simulink model "case5"  (R2024b)
settings: Solver=FixedStepAuto  StartTime=0  StopTime=1  FixedStep=1e-7  RelTol=1e-3
values from neighbouring files (symbols this model uses):
  SG_D_1_D = 0.01056    [IEEE9_case_parameters.m]    (also in case1_parameters.m; case2_parameters.m; case3_parameters.m; case4_parameters.m)
  SG_D_1_EnableSaturation = 0    [IEEE9_case_parameters.m]    (also in case1_parameters.m; case2_parameters.m; case3_parameters.m; case4_parameters.m)
  SG_D_1_f0 = 60    [IEEE9_case_parameters.m]    (also in case1_parameters.m; case2_parameters.m; case3_parameters.m; case4_parameters.m)
  SG_D_1_H = 7.5    [IEEE9_case_parameters.m]    (also in case1_parameters.m; case2_parameters.m; case3_parameters.m; case4_parameters.m)
  SG_D_1_K_A = 20    [IEEE9_case_parameters.m]    (also in case1_parameters.m; case2_parameters.m; case3_parameters.m; case4_parameters.m)
  SG_D_1_K_E = 1.000000e+1    (= 10)    [IEEE9_case_parameters.m]    (also in case1_parameters.m; case2_parameters.m; case3_parameters.m; case4_parameters.m)
  SG_D_1_K_F = 2.363    [IEEE9_case_parameters.m]    (also in case1_parameters.m; case2_parameters.m; case3_parameters.m; case4_parameters.m)
  SG_D_1_K_s = 0.5    [IEEE9_case_parameters.m]    (also in case1_parameters.m = 5; case2_parameters.m = 5; case3_parameters.m = 5; case4_parameters.m = 5)
  SG_D_1_R_a = 0.001088    [IEEE9_case_parameters.m]    (also in case1_parameters.m; case2_parameters.m; case3_parameters.m; case4_parameters.m)
  SG_D_1_S_A = 1    [IEEE9_case_parameters.m]    (also in case1_parameters.m; case2_parameters.m; case3_parameters.m; case4_parameters.m)
  SG_D_1_S_B = 0.103    [IEEE9_case_parameters.m]    (also in case1_parameters.m; case2_parameters.m; case3_parameters.m; case4_parameters.m)
  SG_D_1_S_N = 10.659857    [IEEE9_case_parameters.m]    (also in case1_parameters.m; case2_parameters.m; case3_parameters.m; case4_parameters.m)
  SG_D_1_SpeedPara = 200    [IEEE9_case_parameters.m]    (also in case1_parameters.m; case2_parameters.m; case3_parameters.m; case4_parameters.m)
  SG_D_1_T_0 = 0.720173    [IEEE9_case_parameters.m]    (also in case1_parameters.m = 0.755522; case2_parameters.m = 0.808931; case3_parameters.m = 0.869402; case4_parameters.m = 0.729316)
  SG_D_1_T_1 = 0.3    [IEEE9_case_parameters.m]    (also in case1_parameters.m; case2_parameters.m; case3_parameters.m; case4_parameters.m)
  SG_D_1_T_2 = 0.05    [IEEE9_case_parameters.m]    (also in case1_parameters.m; case2_parameters.m; case3_parameters.m; case4_parameters.m)
  SG_D_1_T_3 = 0.02    [IEEE9_case_parameters.m]    (also in case1_parameters.m; case2_parameters.m; case3_parameters.m; case4_parameters.m)
  SG_D_1_T_4 = 0.005    [IEEE9_case_parameters.m]    (also in case1_parameters.m; case2_parameters.m; case3_parameters.m; case4_parameters.m)
  SG_D_1_T_A = 0.02    [IEEE9_case_parameters.m]    (also in case1_parameters.m; case2_parameters.m; case3_parameters.m; case4_parameters.m)
  SG_D_1_T_dd = 8.000000e+0    (= 8)    [IEEE9_case_parameters.m]    (also in case1_parameters.m; case2_parameters.m; case3_parameters.m; case4_parameters.m)
  SG_D_1_T_ddd = 0.04    [IEEE9_case_parameters.m]    (also in case1_parameters.m; case2_parameters.m; case3_parameters.m; case4_parameters.m)
  SG_D_1_T_E = 0.314    [IEEE9_case_parameters.m]    (also in case1_parameters.m; case2_parameters.m; case3_parameters.m; case4_parameters.m)
  SG_D_1_T_F = 0.35    [IEEE9_case_parameters.m]    (also in case1_parameters.m; case2_parameters.m; case3_parameters.m; case4_parameters.m)
  SG_D_1_T_qd = 0.8    [IEEE9_case_parameters.m]    (also in case1_parameters.m; case2_parameters.m; case3_parameters.m; case4_parameters.m)
  SG_D_1_T_qdd = 0.02    [IEEE9_case_parameters.m]    (also in case1_parameters.m; case2_parameters.m; case3_parameters.m; case4_parameters.m)
  SG_D_1_T_speed = 0.1    [IEEE9_case_parameters.m]    (also in case1_parameters.m = 200; case2_parameters.m = 200; case3_parameters.m = 200; case4_parameters.m = 200)
  SG_D_1_T_w = 0.5    [IEEE9_case_parameters.m]    (also in case1_parameters.m; case2_parameters.m; case3_parameters.m; case4_parameters.m)
  SG_D_1_V_ref = 1.990276    [IEEE9_case_parameters.m]    (also in case1_parameters.m = 2.042296; case2_parameters.m = 2.051388; case3_parameters.m = 2.089584; case4_parameters.m = 2.01845)
  SG_D_1_w_ref = 376.991118    [IEEE9_case_parameters.m]    (also in case1_parameters.m; case2_parameters.m; case3_parameters.m; case4_parameters.m)
  SG_D_1_wb = 6.000000e+1    (= 60)    [IEEE9_case_parameters.m]    (also in case1_parameters.m; case2_parameters.m; case3_parameters.m; case4_parameters.m)
  SG_D_1_x_d = 1.9    [IEEE9_case_parameters.m]    (also in case1_parameters.m; case2_parameters.m; case3_parameters.m; case4_parameters.m)
  SG_D_1_x_dd = 0.302    [IEEE9_case_parameters.m]    (also in case1_parameters.m; case2_parameters.m; case3_parameters.m; case4_parameters.m)
  SG_D_1_x_ddd = 0.204    [IEEE9_case_parameters.m]    (also in case1_parameters.m; case2_parameters.m; case3_parameters.m; case4_parameters.m)
  SG_D_1_x_l = 0.05    [IEEE9_case_parameters.m]    (also in case1_parameters.m; case2_parameters.m; case3_parameters.m; case4_parameters.m)
  SG_D_1_x_q = 1.3    [IEEE9_case_parameters.m]    (also in case1_parameters.m; case2_parameters.m; case3_parameters.m; case4_parameters.m)
  SG_D_1_x_qd = 0.5    [IEEE9_case_parameters.m]    (also in case1_parameters.m; case2_parameters.m; case3_parameters.m; case4_parameters.m)
  SG_D_1_x_qdd = 0.3    [IEEE9_case_parameters.m]    (also in case1_parameters.m; case2_parameters.m; case3_parameters.m; case4_parameters.m)
  SG_D_2_D = 0.02    [IEEE9_case_parameters.m]    (also in case1_parameters.m; case2_parameters.m; case3_parameters.m; case4_parameters.m)
  SG_D_2_EnableSaturation = 0    [IEEE9_case_parameters.m]    (also in case1_parameters.m; case2_parameters.m; case3_parameters.m; case4_parameters.m)
  SG_D_2_f0 = 60    [IEEE9_case_parameters.m]    (also in case1_parameters.m; case2_parameters.m; case3_parameters.m; case4_parameters.m)
  SG_D_2_H = 8.000000e+0    (= 8)    [IEEE9_case_parameters.m]    (also in case1_parameters.m; case2_parameters.m; case3_parameters.m; case4_parameters.m)
  SG_D_2_K_A = 20    [IEEE9_case_parameters.m]    (also in case1_parameters.m; case2_parameters.m; case3_parameters.m; case4_parameters.m)
  SG_D_2_K_E = 1.000000e+1    (= 10)    [IEEE9_case_parameters.m]    (also in case1_parameters.m; case2_parameters.m; case3_parameters.m; case4_parameters.m)
  SG_D_2_K_F = 2.363    [IEEE9_case_parameters.m]    (also in case1_parameters.m; case2_parameters.m; case3_parameters.m; case4_parameters.m)
  SG_D_2_K_s = 0.5    [IEEE9_case_parameters.m]    (also in case1_parameters.m = 4; case2_parameters.m = 4; case3_parameters.m = 4; case4_parameters.m = 4)
  SG_D_2_R_a = 0.001088    [IEEE9_case_parameters.m]    (also in case1_parameters.m; case2_parameters.m; case3_parameters.m; case4_parameters.m)
  SG_D_2_S_A = 1    [IEEE9_case_parameters.m]    (also in case1_parameters.m; case2_parameters.m; case3_parameters.m; case4_parameters.m)
  SG_D_2_S_B = 0.103    [IEEE9_case_parameters.m]    (also in case1_parameters.m; case2_parameters.m; case3_parameters.m; case4_parameters.m)
  SG_D_2_S_N = 10.659857    [IEEE9_case_parameters.m]    (also in case1_parameters.m; case2_parameters.m; case3_parameters.m; case4_parameters.m)
  SG_D_2_SpeedPara = 200    [IEEE9_case_parameters.m]    (also in case1_parameters.m; case2_parameters.m; case3_parameters.m; case4_parameters.m)
  SG_D_2_T_0 = 1.632913    [IEEE9_case_parameters.m]    (also in case1_parameters.m = 1.632925; case2_parameters.m = 1.632915; case3_parameters.m = 1.632914; case4_parameters.m = 1.632927)
  SG_D_2_T_1 = 0.2    [IEEE9_case_parameters.m]    (also in case1_parameters.m; case2_parameters.m; case3_parameters.m; case4_parameters.m)
  SG_D_2_T_2 = 0.05    [IEEE9_case_parameters.m]    (also in case1_parameters.m; case2_parameters.m; case3_parameters.m; case4_parameters.m)
  SG_D_2_T_3 = 0.02    [IEEE9_case_parameters.m]    (also in case1_parameters.m; case2_parameters.m; case3_parameters.m; case4_parameters.m)
  SG_D_2_T_4 = 0.005    [IEEE9_case_parameters.m]    (also in case1_parameters.m; case2_parameters.m; case3_parameters.m; case4_parameters.m)
  SG_D_2_T_A = 0.02    [IEEE9_case_parameters.m]    (also in case1_parameters.m; case2_parameters.m; case3_parameters.m; case4_parameters.m)
  SG_D_2_T_dd = 7.9    [IEEE9_case_parameters.m]    (also in case1_parameters.m; case2_parameters.m; case3_parameters.m; case4_parameters.m)
  SG_D_2_T_ddd = 0.04    [IEEE9_case_parameters.m]    (also in case1_parameters.m; case2_parameters.m; case3_parameters.m; case4_parameters.m)
  SG_D_2_T_E = 0.314    [IEEE9_case_parameters.m]    (also in case1_parameters.m; case2_parameters.m; case3_parameters.m; case4_parameters.m)
  SG_D_2_T_F = 0.35    [IEEE9_case_parameters.m]    (also in case1_parameters.m; case2_parameters.m; case3_parameters.m; case4_parameters.m)
  SG_D_2_T_qd = 0.8    [IEEE9_case_parameters.m]    (also in case1_parameters.m; case2_parameters.m; case3_parameters.m; case4_parameters.m)
  SG_D_2_T_qdd = 0.015    [IEEE9_case_parameters.m]    (also in case1_parameters.m; case2_parameters.m; case3_parameters.m; case4_parameters.m)
  SG_D_2_T_speed = 0.1    [IEEE9_case_parameters.m]    (also in case1_parameters.m = 150; case2_parameters.m = 150; case3_parameters.m = 150; case4_parameters.m = 150)
  SG_D_2_T_w = 0.35    [IEEE9_case_parameters.m]    (also in case1_parameters.m; case2_parameters.m; case3_parameters.m; case4_parameters.m)
  SG_D_2_V_ref = 2.58547    [IEEE9_case_parameters.m]    (also in case1_parameters.m = 2.597896; case2_parameters.m = 2.587136; case3_parameters.m = 2.586042; case4_parameters.m = 2.599679)
  SG_D_2_w_ref = 376.991118    [IEEE9_case_parameters.m]    (also in case1_parameters.m; case2_parameters.m; case3_parameters.m; case4_parameters.m)
  SG_D_2_wb = 6.000000e+1    (= 60)    [IEEE9_case_parameters.m]    (also in case1_parameters.m; case2_parameters.m; case3_parameters.m; case4_parameters.m)
  SG_D_2_x_d = 1.8    [IEEE9_case_parameters.m]    (also in case1_parameters.m; case2_parameters.m; case3_parameters.m; case4_parameters.m)
  SG_D_2_x_dd = 0.302    [IEEE9_case_parameters.m]    (also in case1_parameters.m; case2_parameters.m; case3_parameters.m; case4_parameters.m)
  SG_D_2_x_ddd = 0.204    [IEEE9_case_parameters.m]    (also in case1_parameters.m; case2_parameters.m; case3_parameters.m; case4_parameters.m)
  SG_D_2_x_l = 0.05    [IEEE9_case_parameters.m]    (also in case1_parameters.m; case2_parameters.m; case3_parameters.m; case4_parameters.m)
  SG_D_2_x_q = 1.25    [IEEE9_case_parameters.m]    (also in case1_parameters.m; case2_parameters.m; case3_parameters.m; case4_parameters.m)
  SG_D_2_x_qd = 0.5    [IEEE9_case_parameters.m]    (also in case1_parameters.m; case2_parameters.m; case3_parameters.m; case4_parameters.m)
  SG_D_2_x_qdd = 0.3    [IEEE9_case_parameters.m]    (also in case1_parameters.m; case2_parameters.m; case3_parameters.m; case4_parameters.m)
  SG_D_3_D = 0.02    [IEEE9_case_parameters.m]    (also in case1_parameters.m; case2_parameters.m; case3_parameters.m; case4_parameters.m)
  SG_D_3_EnableSaturation = 0    [IEEE9_case_parameters.m]    (also in case1_parameters.m; case2_parameters.m; case3_parameters.m; case4_parameters.m)
  SG_D_3_f0 = 60    [IEEE9_case_parameters.m]    (also in case1_parameters.m; case2_parameters.m; case3_parameters.m; case4_parameters.m)
  SG_D_3_H = 7.7    [IEEE9_case_parameters.m]    (also in case1_parameters.m; case2_parameters.m; case3_parameters.m; case4_parameters.m)
  SG_D_3_K_A = 20    [IEEE9_case_parameters.m]    (also in case1_parameters.m; case2_parameters.m; case3_parameters.m; case4_parameters.m)
  SG_D_3_K_E = 1.000000e+1    (= 10)    [IEEE9_case_parameters.m]    (also in case1_parameters.m; case2_parameters.m; case3_parameters.m; case4_parameters.m)
  SG_D_3_K_F = 2.363    [IEEE9_case_parameters.m]    (also in case1_parameters.m; case2_parameters.m; case3_parameters.m; case4_parameters.m)
  SG_D_3_K_s = 0.2    [IEEE9_case_parameters.m]    (also in case1_parameters.m = 2; case2_parameters.m = 2; case3_parameters.m = 2; case4_parameters.m = 2)
  SG_D_3_R_a = 0.001088    [IEEE9_case_parameters.m]    (also in case1_parameters.m; case2_parameters.m; case3_parameters.m; case4_parameters.m)
  SG_D_3_S_A = 1    [IEEE9_case_parameters.m]    (also in case1_parameters.m; case2_parameters.m; case3_parameters.m; case4_parameters.m)
  SG_D_3_S_B = 0.103    [IEEE9_case_parameters.m]    (also in case1_parameters.m; case2_parameters.m; case3_parameters.m; case4_parameters.m)
  SG_D_3_S_N = 10.659857    [IEEE9_case_parameters.m]    (also in case1_parameters.m; case2_parameters.m; case3_parameters.m; case4_parameters.m)
  SG_D_3_SpeedPara = 200    [IEEE9_case_parameters.m]    (also in case1_parameters.m; case2_parameters.m; case3_parameters.m; case4_parameters.m)
  SG_D_3_T_0 = 0.850788    [IEEE9_case_parameters.m]    (also in case1_parameters.m = 0.850786; case2_parameters.m = 0.850787; case3_parameters.m; case4_parameters.m = 0.850786)
  SG_D_3_T_1 = 0.2    [IEEE9_case_parameters.m]    (also in case1_parameters.m; case2_parameters.m; case3_parameters.m; case4_parameters.m)
  SG_D_3_T_2 = 0.05    [IEEE9_case_parameters.m]    (also in case1_parameters.m; case2_parameters.m; case3_parameters.m; case4_parameters.m)
  SG_D_3_T_3 = 0.02    [IEEE9_case_parameters.m]    (also in case1_parameters.m; case2_parameters.m; case3_parameters.m; case4_parameters.m)
  SG_D_3_T_4 = 0.005    [IEEE9_case_parameters.m]    (also in case1_parameters.m; case2_parameters.m; case3_parameters.m; case4_parameters.m)
  SG_D_3_T_A = 0.02    [IEEE9_case_parameters.m]    (also in case1_parameters.m; case2_parameters.m; case3_parameters.m; case4_parameters.m)
  SG_D_3_T_dd = 8.1    [IEEE9_case_parameters.m]    (also in case1_parameters.m; case2_parameters.m; case3_parameters.m; case4_parameters.m)
  SG_D_3_T_ddd = 0.04    [IEEE9_case_parameters.m]    (also in case1_parameters.m; case2_parameters.m; case3_parameters.m; case4_parameters.m)
  SG_D_3_T_E = 0.314    [IEEE9_case_parameters.m]    (also in case1_parameters.m; case2_parameters.m; case3_parameters.m; case4_parameters.m)
  SG_D_3_T_F = 0.35    [IEEE9_case_parameters.m]    (also in case1_parameters.m; case2_parameters.m; case3_parameters.m; case4_parameters.m)
  SG_D_3_T_qd = 0.8    [IEEE9_case_parameters.m]    (also in case1_parameters.m; case2_parameters.m; case3_parameters.m; case4_parameters.m)
  SG_D_3_T_qdd = 0.015    [IEEE9_case_parameters.m]    (also in case1_parameters.m; case2_parameters.m; case3_parameters.m; case4_parameters.m)
  SG_D_3_T_speed = 0.1    [IEEE9_case_parameters.m]    (also in case1_parameters.m = 180; case2_parameters.m = 180; case3_parameters.m = 180; case4_parameters.m = 180)
  SG_D_3_T_w = 0.4    [IEEE9_case_parameters.m]    (also in case1_parameters.m; case2_parameters.m; case3_parameters.m; case4_parameters.m)
  SG_D_3_V_ref = 1.892727    [IEEE9_case_parameters.m]    (also in case1_parameters.m = 1.906439; case2_parameters.m = 1.895535; case3_parameters.m = 1.892105; case4_parameters.m = 1.906598)
  SG_D_3_w_ref = 376.991118    [IEEE9_case_parameters.m]    (also in case1_parameters.m; case2_parameters.m; case3_parameters.m; case4_parameters.m)
  SG_D_3_wb = 6.000000e+1    (= 60)    [IEEE9_case_parameters.m]    (also in case1_parameters.m; case2_parameters.m; case3_parameters.m; case4_parameters.m)
  SG_D_3_x_d = 1.85    [IEEE9_case_parameters.m]    (also in case1_parameters.m; case2_parameters.m; case3_parameters.m; case4_parameters.m)
  SG_D_3_x_dd = 0.302    [IEEE9_case_parameters.m]    (also in case1_parameters.m; case2_parameters.m; case3_parameters.m; case4_parameters.m)
  SG_D_3_x_ddd = 0.204    [IEEE9_case_parameters.m]    (also in case1_parameters.m; case2_parameters.m; case3_parameters.m; case4_parameters.m)
  SG_D_3_x_l = 0.05    [IEEE9_case_parameters.m]    (also in case1_parameters.m; case2_parameters.m; case3_parameters.m; case4_parameters.m)
  SG_D_3_x_q = 1.2    [IEEE9_case_parameters.m]    (also in case1_parameters.m; case2_parameters.m; case3_parameters.m; case4_parameters.m)
  SG_D_3_x_qd = 0.5    [IEEE9_case_parameters.m]    (also in case1_parameters.m; case2_parameters.m; case3_parameters.m; case4_parameters.m)
  SG_D_3_x_qdd = 0.3    [IEEE9_case_parameters.m]    (also in case1_parameters.m; case2_parameters.m; case3_parameters.m; case4_parameters.m)
(part 3 of 12)

== system case5/AC_1/d_id_load_7_block ==
  note: d_id_load_7 in case5
      | $376.991118430775\,\mathrm{iq}_{\mathrm{load},7}-1031.50171752067\,\mathrm{id}_{\mathrm{load},7}+1182.0806386337\,\mathrm{vd}_{\mathrm{bus},7}$
      | Automatically generated on 2025-10-31 19:14:07 .
  State_id_load_7_b98f0 : Inport
  State_iq_load_7_60963 : Inport  Port=2
  State_vd_bus_7_34461 : Inport  Port=3
  Add_5da86 : Sum
  Add_d2ee0 : Sum
  Constant_-1031.50171752067_88356 : Constant  Value=-1031.50171752067
  Constant_1182.0806386337_d4c60 : Constant  Value=1182.0806386337
  Constant_376.991118430775_acd9e : Constant  Value=376.991118430775
  Product_668db : Product
  Product_8018d : Product
  Product_f008c : Product
  Blockout_d_id_load_7_04e2e : Outport
  wires:
  Constant_-1031.50171752067_88356/1 -> Product_f008c/1
  Product_668db/1 -> Add_d2ee0/2
  State_id_load_7_b98f0/1 -> Product_f008c/2
  Constant_376.991118430775_acd9e/1 -> Product_668db/1
  Product_f008c/1 -> Add_d2ee0/1
  State_iq_load_7_60963/1 -> Product_668db/2
  Constant_1182.0806386337_d4c60/1 -> Product_8018d/1
  State_vd_bus_7_34461/1 -> Product_8018d/2
  Add_d2ee0/1 -> Add_5da86/1
  Product_8018d/1 -> Add_5da86/2
  Add_5da86/1 -> Blockout_d_id_load_7_04e2e/1

== system case5/AC_1/d_id_load_9_block ==
  note: d_id_load_9 in case5
      | $376.991118430775\,\mathrm{iq}_{\mathrm{load},9}-902.564002881027\,\mathrm{id}_{\mathrm{load},9}+1422.06408334706\,\mathrm{vd}_{\mathrm{bus},9}$
      | Automatically generated on 2025-10-31 19:14:10 .
  State_id_load_9_852e2 : Inport
  State_iq_load_9_0074f : Inport  Port=2
  State_vd_bus_9_ae388 : Inport  Port=3
  Add_87244 : Sum
  Add_a625d : Sum
  Constant_-902.564002881027_5e5dd : Constant  Value=-902.564002881027
  Constant_1422.06408334706_f4d59 : Constant  Value=1422.06408334706
  Constant_376.991118430775_c11f6 : Constant  Value=376.991118430775
  Product_527e2 : Product
  Product_9fd9e : Product
  Product_b3dcd : Product
  Blockout_d_id_load_9_1c904 : Outport
  wires:
  Constant_-902.564002881027_5e5dd/1 -> Product_527e2/1
  Product_b3dcd/1 -> Add_87244/2
  State_id_load_9_852e2/1 -> Product_527e2/2
  Constant_376.991118430775_c11f6/1 -> Product_b3dcd/1
  Product_527e2/1 -> Add_87244/1
  State_iq_load_9_0074f/1 -> Product_b3dcd/2
  Constant_1422.06408334706_f4d59/1 -> Product_9fd9e/1
  State_vd_bus_9_ae388/1 -> Product_9fd9e/2
  Add_87244/1 -> Add_a625d/1
  Product_9fd9e/1 -> Add_a625d/2
  Add_a625d/1 -> Blockout_d_id_load_9_1c904/1

== system case5/AC_1/d_iq_line_1_4_block ==
  note: d_iq_line_1_4 in case5
      | $6332.81249201072\,\mathrm{vq}_{\mathrm{bus},1}-376.991118430775\,\mathrm{id}_{\mathrm{line},1,4}-6332.81249201072\,\mathrm{vq}_{\mathrm{bus},4}$
      | Automatically generated on 2025-10-31 19:14:14 .
  State_id_line_1_4_b0e34 : Inport
  State_vq_bus_1_10e2e : Inport  Port=2
  State_vq_bus_4_12e2c : Inport  Port=3
  Add_ee68b : Sum
  Constant_-376.991118430775_981b4 : Constant  Value=-376.991118430775
  Constant_6332.81249201072_4ba04 : Constant  Value=6332.81249201072
  Constant_6332.81249201072_e276d : Constant  Value=6332.81249201072
  Product_09aeb : Product
  Product_22e0f : Product
  Product_35656 : Product
  Subtract_01ad3 : Sum  Inputs=+-
  Blockout_d_iq_line_1_4_2dd06 : Outport
  wires:
  Constant_-376.991118430775_981b4/1 -> Product_35656/1
  Product_22e0f/1 -> Add_ee68b/2
  State_id_line_1_4_b0e34/1 -> Product_35656/2
  Constant_6332.81249201072_4ba04/1 -> Product_22e0f/1
  Product_35656/1 -> Add_ee68b/1
  Subtract_01ad3/1 -> Blockout_d_iq_line_1_4_2dd06/1
  State_vq_bus_1_10e2e/1 -> Product_22e0f/2
  Constant_6332.81249201072_e276d/1 -> Product_09aeb/1
  State_vq_bus_4_12e2c/1 -> Product_09aeb/2
  Add_ee68b/1 -> Subtract_01ad3/1
  Product_09aeb/1 -> Subtract_01ad3/2

== system case5/AC_1/d_iq_line_3_6_block ==
  note: d_iq_line_3_6 in case5
      | $6224.74401945081\,\mathrm{vq}_{\mathrm{bus},3}-376.991118430775\,\mathrm{id}_{\mathrm{line},3,6}-6224.74401945081\,\mathrm{vq}_{\mathrm{bus},6}$
      | Automatically generated on 2025-10-31 19:14:24 .
  State_id_line_3_6_990b7 : Inport
  State_vq_bus_3_aba8c : Inport  Port=2
  State_vq_bus_6_39c16 : Inport  Port=3
  Add_ffe2b : Sum
  Constant_-376.991118430775_48885 : Constant  Value=-376.991118430775
  Constant_6224.74401945081_5858a : Constant  Value=6224.74401945081
  Constant_6224.74401945081_c535b : Constant  Value=6224.74401945081
  Product_030a8 : Product
  Product_915a9 : Product
  Product_beaa7 : Product
  Subtract_94097 : Sum  Inputs=+-
  Blockout_d_iq_line_3_6_60ca3 : Outport
  wires:
  Constant_-376.991118430775_48885/1 -> Product_915a9/1
  Product_beaa7/1 -> Add_ffe2b/2
  State_id_line_3_6_990b7/1 -> Product_915a9/2
  Constant_6224.74401945081_5858a/1 -> Product_beaa7/1
  Product_915a9/1 -> Add_ffe2b/1
  State_vq_bus_3_aba8c/1 -> Product_beaa7/2
  Constant_6224.74401945081_c535b/1 -> Product_030a8/1
  State_vq_bus_6_39c16/1 -> Product_030a8/2
  Add_ffe2b/1 -> Subtract_94097/1
  Product_030a8/1 -> Subtract_94097/2
  Subtract_94097/1 -> Blockout_d_iq_line_3_6_60ca3/1

== system case5/AC_1/d_iq_line_4_5_block ==
  note: d_iq_line_4_5 in case5
      | $3964.89129934584\,\mathrm{vq}_{\mathrm{bus},4}-65.6746171008477\,\mathrm{iq}_{\mathrm{line},4,5}-376.991118430775\,\mathrm{id}_{\mathrm{line},4,5}-3964.89129934584\,\mathrm{vq}_{\mathrm{bus},5}$
      | Automatically generated on 2025-10-31 19:14:18 .
  State_id_line_4_5_5fe62 : Inport
  State_iq_line_4_5_78122 : Inport  Port=2
  State_vq_bus_4_7d2aa : Inport  Port=3
  State_vq_bus_5_c2555 : Inport  Port=4
  Add_26ea8 : Sum
  Constant_-376.991118430775_ffbcc : Constant  Value=-376.991118430775
  Constant_3964.89129934584_2fa91 : Constant  Value=3964.89129934584
  Constant_3964.89129934584_db51c : Constant  Value=3964.89129934584
  Constant_65.6746171008477_cc033 : Constant  Value=65.6746171008477
  Product_7fe87 : Product
  Product_99dad : Product
  Product_a7fd6 : Product
  Product_fe884 : Product
  Subtract_6d03a : Sum  Inputs=+-
  Subtract_75c15 : Sum  Inputs=+-
  Blockout_d_iq_line_4_5_957bf : Outport
  wires:
  Constant_-376.991118430775_ffbcc/1 -> Product_99dad/1
  Constant_65.6746171008477_cc033/1 -> Product_a7fd6/1
  State_id_line_4_5_5fe62/1 -> Product_99dad/2
  State_iq_line_4_5_78122/1 -> Product_a7fd6/2
  Product_99dad/1 -> Subtract_6d03a/1
  Constant_3964.89129934584_db51c/1 -> Product_fe884/1
  Product_a7fd6/1 -> Subtract_6d03a/2
  State_vq_bus_4_7d2aa/1 -> Product_fe884/2
  Subtract_6d03a/1 -> Add_26ea8/1
  Product_fe884/1 -> Add_26ea8/2
  Constant_3964.89129934584_2fa91/1 -> Product_7fe87/1
  State_vq_bus_5_c2555/1 -> Product_7fe87/2
  Add_26ea8/1 -> Subtract_75c15/1
  Product_7fe87/1 -> Subtract_75c15/2
  Subtract_75c15/1 -> Blockout_d_iq_line_4_5_957bf/1

== system case5/AC_1/d_iq_line_5_6_block ==
  note: d_iq_line_5_6 in case5
      | $2145.70587964598\,\mathrm{vq}_{\mathrm{bus},5}-81.5365142414676\,\mathrm{iq}_{\mathrm{line},5,6}-376.991118430775\,\mathrm{id}_{\mathrm{line},5,6}-2145.70587964598\,\mathrm{vq}_{\mathrm{bus},6}$
      | Automatically generated on 2025-10-31 19:14:21 .
  State_id_line_5_6_8cff1 : Inport
  State_iq_line_5_6_03329 : Inport  Port=2
  State_vq_bus_5_a71a3 : Inport  Port=3
  State_vq_bus_6_551df : Inport  Port=4
  Add_62605 : Sum
  Constant_-376.991118430775_01fb4 : Constant  Value=-376.991118430775
  Constant_2145.70587964598_b21ee : Constant  Value=2145.70587964598
  Constant_2145.70587964598_ff72d : Constant  Value=2145.70587964598
  Constant_81.5365142414676_e1a8f : Constant  Value=81.5365142414676
  Product_a6071 : Product
  Product_ab8bb : Product
  Product_b8793 : Product
  Product_f3c1e : Product
  Subtract_0b3f6 : Sum  Inputs=+-
  Subtract_3a87d : Sum  Inputs=+-
  Blockout_d_iq_line_5_6_5852f : Outport
  wires:
  Constant_-376.991118430775_01fb4/1 -> Product_ab8bb/1
  Constant_81.5365142414676_e1a8f/1 -> Product_a6071/1
  Subtract_0b3f6/1 -> Blockout_d_iq_line_5_6_5852f/1
  State_id_line_5_6_8cff1/1 -> Product_ab8bb/2
  State_iq_line_5_6_03329/1 -> Product_a6071/2
  Product_ab8bb/1 -> Subtract_3a87d/1
  Constant_2145.70587964598_b21ee/1 -> Product_b8793/1
  Product_a6071/1 -> Subtract_3a87d/2
  Product_f3c1e/1 -> Subtract_0b3f6/2
  State_vq_bus_5_a71a3/1 -> Product_b8793/2
  Subtract_3a87d/1 -> Add_62605/1
  Product_b8793/1 -> Add_62605/2
  Constant_2145.70587964598_ff72d/1 -> Product_f3c1e/1
  State_vq_bus_6_551df/1 -> Product_f3c1e/2
  Add_62605/1 -> Subtract_0b3f6/1

== system case5/AC_1/d_iq_line_6_7_block ==
  note: d_iq_line_6_7 in case5
      | $3618.7499954347\,\mathrm{vq}_{\mathrm{bus},6}-41.9587831477638\,\mathrm{iq}_{\mathrm{line},6,7}-376.991118430775\,\mathrm{id}_{\mathrm{line},6,7}-3618.7499954347\,\mathrm{vq}_{\mathrm{bus},7}$
      | Automatically generated on 2025-10-31 19:14:28 .
  State_id_line_6_7_0d433 : Inport
  State_iq_line_6_7_8faef : Inport  Port=2
  State_vq_bus_6_4ace9 : Inport  Port=3
  State_vq_bus_7_fbcef : Inport  Port=4
  Add_5ed2d : Sum
  Constant_-376.991118430775_26131 : Constant  Value=-376.991118430775
  Constant_3618.7499954347_23295 : Constant  Value=3618.7499954347
  Constant_3618.7499954347_90f0d : Constant  Value=3618.7499954347
  Constant_41.9587831477638_9583f : Constant  Value=41.9587831477638
  Product_0d19f : Product
  Product_23081 : Product
  Product_37f12 : Product
  Product_af732 : Product
  Subtract_6f523 : Sum  Inputs=+-
  Subtract_8b9bd : Sum  Inputs=+-
  Blockout_d_iq_line_6_7_67cbf : Outport
  wires:
  Constant_-376.991118430775_26131/1 -> Product_af732/1
  Constant_41.9587831477638_9583f/1 -> Product_37f12/1
  State_id_line_6_7_0d433/1 -> Product_af732/2
  State_iq_line_6_7_8faef/1 -> Product_37f12/2
  Product_af732/1 -> Subtract_8b9bd/1
  Constant_3618.7499954347_23295/1 -> Product_23081/1
  Product_37f12/1 -> Subtract_8b9bd/2
  State_vq_bus_6_4ace9/1 -> Product_23081/2
  Subtract_8b9bd/1 -> Add_5ed2d/1
  Product_23081/1 -> Add_5ed2d/2
  Constant_3618.7499954347_90f0d/1 -> Product_0d19f/1
  State_vq_bus_7_fbcef/1 -> Product_0d19f/2
  Add_5ed2d/1 -> Subtract_6f523/1
  Product_0d19f/1 -> Subtract_6f523/2
  Subtract_6f523/1 -> Blockout_d_iq_line_6_7_67cbf/1

== system case5/AC_1/d_iq_line_7_8_block ==
  note: d_iq_line_7_8 in case5
      | $5066.24999360857\,\mathrm{vq}_{\mathrm{bus},7}-41.9587831477638\,\mathrm{iq}_{\mathrm{line},7,8}-376.991118430775\,\mathrm{id}_{\mathrm{line},7,8}-5066.24999360857\,\mathrm{vq}_{\mathrm{bus},8}$
      | Automatically generated on 2025-10-31 19:14:31 .
  State_id_line_7_8_196fb : Inport
  State_iq_line_7_8_38443 : Inport  Port=2
  State_vq_bus_7_6977a : Inport  Port=3
  State_vq_bus_8_202ba : Inport  Port=4
  Add_8acf1 : Sum
  Constant_-376.991118430775_a2955 : Constant  Value=-376.991118430775
  Constant_41.9587831477638_8785a : Constant  Value=41.9587831477638
  Constant_5066.24999360857_2f997 : Constant  Value=5066.24999360857
  Constant_5066.24999360857_e7552 : Constant  Value=5066.24999360857
  Product_01e47 : Product
  Product_164e5 : Product
  Product_a032e : Product
  Product_deac0 : Product
  Subtract_46a22 : Sum  Inputs=+-
  Subtract_7025c : Sum  Inputs=+-
  Blockout_d_iq_line_7_8_896d8 : Outport
  wires:
  Constant_-376.991118430775_a2955/1 -> Product_deac0/1
  Constant_41.9587831477638_8785a/1 -> Product_a032e/1
  State_id_line_7_8_196fb/1 -> Product_deac0/2
  State_iq_line_7_8_38443/1 -> Product_a032e/2
  Product_deac0/1 -> Subtract_46a22/1
  Constant_5066.24999360857_e7552/1 -> Product_01e47/1
  Product_a032e/1 -> Subtract_46a22/2
  State_vq_bus_7_6977a/1 -> Product_01e47/2
  Subtract_46a22/1 -> Add_8acf1/1
  Product_01e47/1 -> Add_8acf1/2
  Constant_5066.24999360857_2f997/1 -> Product_164e5/1
  State_vq_bus_8_202ba/1 -> Product_164e5/2
  Add_8acf1/1 -> Subtract_7025c/1
  Product_164e5/1 -> Subtract_7025c/2
  Subtract_7025c/1 -> Blockout_d_iq_line_7_8_896d8/1

== system case5/AC_1/d_iq_line_8_2_block ==
  note: d_iq_line_8_2 in case5
      | $5836.31999263708\,\mathrm{vq}_{\mathrm{bus},8}-5836.31999263708\,\mathrm{vq}_{\mathrm{bus},2}-376.991118430775\,\mathrm{id}_{\mathrm{line},8,2}$
      | Automatically generated on 2025-10-31 19:14:35 .
  State_id_line_8_2_763ed : Inport
  State_vq_bus_2_a450a : Inport  Port=2
  State_vq_bus_8_a1826 : Inport  Port=3
  Add_a0022 : Sum
  Constant_-376.991118430775_f3e28 : Constant  Value=-376.991118430775
  Constant_5836.31999263708_07cb9 : Constant  Value=5836.31999263708
  Constant_5836.31999263708_30efe : Constant  Value=5836.31999263708
  Product_2bbb6 : Product
  Product_746ef : Product
  Product_d74a4 : Product
  Subtract_77c5c : Sum  Inputs=+-
  Blockout_d_iq_line_8_2_50cf1 : Outport
  wires:
  Constant_-376.991118430775_f3e28/1 -> Product_d74a4/1
  Product_2bbb6/1 -> Subtract_77c5c/2
  State_id_line_8_2_763ed/1 -> Product_d74a4/2
  Constant_5836.31999263708_30efe/1 -> Product_2bbb6/1
  Product_d74a4/1 -> Subtract_77c5c/1
  State_vq_bus_2_a450a/1 -> Product_2bbb6/2
  Constant_5836.31999263708_07cb9/1 -> Product_746ef/1
  State_vq_bus_8_a1826/1 -> Product_746ef/2
  Subtract_77c5c/1 -> Add_a0022/1
  Product_746ef/1 -> Add_a0022/2
  Add_a0022/1 -> Blockout_d_iq_line_8_2_50cf1/1

== system case5/AC_1/d_iq_line_8_9_block ==
  note: d_iq_line_8_9 in case5
      | $2265.65217105477\,\mathrm{vq}_{\mathrm{bus},8}-70.6416049488109\,\mathrm{iq}_{\mathrm{line},8,9}-376.991118430775\,\mathrm{id}_{\mathrm{line},8,9}-2265.65217105477\,\mathrm{vq}_{\mathrm{bus},9}$
      | Automatically generated on 2025-10-31 19:14:38 .
  State_id_line_8_9_666cc : Inport
  State_iq_line_8_9_bc607 : Inport  Port=2
  State_vq_bus_8_b13ad : Inport  Port=3
  State_vq_bus_9_0596d : Inport  Port=4
  Add_5d7a6 : Sum
  Constant_-376.991118430775_cd39f : Constant  Value=-376.991118430775
  Constant_2265.65217105477_bb948 : Constant  Value=2265.65217105477
  Constant_2265.65217105477_edd94 : Constant  Value=2265.65217105477
  Constant_70.6416049488109_b4dc1 : Constant  Value=70.6416049488109
  Product_2705d : Product
  Product_4cbb4 : Product
  Product_644a4 : Product
  Product_c4e64 : Product
  Subtract_0b512 : Sum  Inputs=+-
  Subtract_1c170 : Sum  Inputs=+-
  Blockout_d_iq_line_8_9_1ed33 : Outport
  wires:
  Constant_-376.991118430775_cd39f/1 -> Product_2705d/1
  Constant_70.6416049488109_b4dc1/1 -> Product_644a4/1
  State_id_line_8_9_666cc/1 -> Product_2705d/2
  State_iq_line_8_9_bc607/1 -> Product_644a4/2
  Product_2705d/1 -> Subtract_0b512/1
  Constant_2265.65217105477_bb948/1 -> Product_4cbb4/1
  Product_644a4/1 -> Subtract_0b512/2
  State_vq_bus_8_b13ad/1 -> Product_4cbb4/2
  Subtract_0b512/1 -> Add_5d7a6/1
  Product_4cbb4/1 -> Add_5d7a6/2
  Constant_2265.65217105477_edd94/1 -> Product_c4e64/1
  Add_5d7a6/1 -> Subtract_1c170/1
  State_vq_bus_9_0596d/1 -> Product_c4e64/2
  Product_c4e64/1 -> Subtract_1c170/2
  Subtract_1c170/1 -> Blockout_d_iq_line_8_9_1ed33/1

== system case5/AC_1/d_iq_line_9_4_block ==
  note: d_iq_line_9_4 in case5
      | $4291.41175929197\,\mathrm{vq}_{\mathrm{bus},9}-41.8135970469065\,\mathrm{iq}_{\mathrm{line},9,4}-4291.41175929197\,\mathrm{vq}_{\mathrm{bus},4}-376.991118430775\,\mathrm{id}_{\mathrm{line},9,4}$
      | Automatically generated on 2025-10-31 19:14:42 .
  State_id_line_9_4_c3c0d : Inport
  State_iq_line_9_4_03835 : Inport  Port=2
  State_vq_bus_4_0a95d : Inport  Port=3
  State_vq_bus_9_291a8 : Inport  Port=4
  Add_c8b14 : Sum
  Constant_-376.991118430775_dbab7 : Constant  Value=-376.991118430775
  Constant_41.8135970469065_329e2 : Constant  Value=41.8135970469065
  Constant_4291.41175929197_22870 : Constant  Value=4291.41175929197
  Constant_4291.41175929197_47bfb : Constant  Value=4291.41175929197
  Product_1e610 : Product
  Product_34c97 : Product
  Product_8063e : Product
  Product_af7a8 : Product
  Subtract_91210 : Sum  Inputs=+-
  Subtract_e3df7 : Sum  Inputs=+-
  Blockout_d_iq_line_9_4_b0247 : Outport
  wires:
  Constant_-376.991118430775_dbab7/1 -> Product_1e610/1
  Constant_41.8135970469065_329e2/1 -> Product_34c97/1
  State_id_line_9_4_c3c0d/1 -> Product_1e610/2
  State_iq_line_9_4_03835/1 -> Product_34c97/2
  Product_1e610/1 -> Subtract_91210/1
  Constant_4291.41175929197_47bfb/1 -> Product_af7a8/1
  Product_34c97/1 -> Subtract_91210/2
  State_vq_bus_4_0a95d/1 -> Product_af7a8/2
  Subtract_91210/1 -> Subtract_e3df7/1
  Product_af7a8/1 -> Subtract_e3df7/2
  Constant_4291.41175929197_22870/1 -> Product_8063e/1
  Add_c8b14/1 -> Blockout_d_iq_line_9_4_b0247/1
  State_vq_bus_9_291a8/1 -> Product_8063e/2
  Subtract_e3df7/1 -> Add_c8b14/1
  Product_8063e/1 -> Add_c8b14/2

== system case5/AC_1/d_iq_load_5_block ==
  note: d_iq_load_5 in case5
      | $1127.5659037617\,\mathrm{vq}_{\mathrm{bus},5}-1083.07680322081\,\mathrm{iq}_{\mathrm{load},5}-376.991118430775\,\mathrm{id}_{\mathrm{load},5}$
      | Automatically generated on 2025-10-31 19:14:05 .
  State_id_load_5_12f97 : Inport
  State_iq_load_5_4667a : Inport  Port=2
  State_vq_bus_5_ae904 : Inport  Port=3
  Add_287f1 : Sum
  Constant_-376.991118430775_ae034 : Constant  Value=-376.991118430775
  Constant_1083.07680322081_eeae4 : Constant  Value=1083.07680322081
  Constant_1127.5659037617_818c2 : Constant  Value=1127.5659037617
  Product_7e0c9 : Product
  Product_9f8d6 : Product
  Product_c7a31 : Product
  Subtract_3840c : Sum  Inputs=+-
  Blockout_d_iq_load_5_ea36b : Outport
  wires:
  Constant_-376.991118430775_ae034/1 -> Product_9f8d6/1
  Product_7e0c9/1 -> Subtract_3840c/2
  State_id_load_5_12f97/1 -> Product_9f8d6/2
  Constant_1083.07680322081_eeae4/1 -> Product_7e0c9/1
  Product_9f8d6/1 -> Subtract_3840c/1
  State_iq_load_5_4667a/1 -> Product_7e0c9/2
  Constant_1127.5659037617_818c2/1 -> Product_c7a31/1
  State_vq_bus_5_ae904/1 -> Product_c7a31/2
  Subtract_3840c/1 -> Add_287f1/1
  Product_c7a31/1 -> Add_287f1/2
  Add_287f1/1 -> Blockout_d_iq_load_5_ea36b/1

== system case5/AC_1/d_iq_load_7_block ==
  note: d_iq_load_7 in case5
      | $1182.0806386337\,\mathrm{vq}_{\mathrm{bus},7}-1031.50171752067\,\mathrm{iq}_{\mathrm{load},7}-376.991118430775\,\mathrm{id}_{\mathrm{load},7}$
      | Automatically generated on 2025-10-31 19:14:08 .
  State_id_load_7_92af4 : Inport
  State_iq_load_7_a25bd : Inport  Port=2
  State_vq_bus_7_b5d78 : Inport  Port=3
  Add_77e8b : Sum
  Constant_-376.991118430775_c40ec : Constant  Value=-376.991118430775
  Constant_1031.50171752067_6da58 : Constant  Value=1031.50171752067
  Constant_1182.0806386337_6074c : Constant  Value=1182.0806386337
  Product_32698 : Product
  Product_743c1 : Product
  Product_f3726 : Product
  Subtract_ba7fa : Sum  Inputs=+-
  Blockout_d_iq_load_7_b7b7d : Outport
  wires:
  Constant_-376.991118430775_c40ec/1 -> Product_743c1/1
  Product_f3726/1 -> Subtract_ba7fa/2
  State_id_load_7_92af4/1 -> Product_743c1/2
  Constant_1031.50171752067_6da58/1 -> Product_f3726/1
  Product_743c1/1 -> Subtract_ba7fa/1
  State_iq_load_7_a25bd/1 -> Product_f3726/2
  Constant_1182.0806386337_6074c/1 -> Product_32698/1
  State_vq_bus_7_b5d78/1 -> Product_32698/2
  Subtract_ba7fa/1 -> Add_77e8b/1
  Product_32698/1 -> Add_77e8b/2
  Add_77e8b/1 -> Blockout_d_iq_load_7_b7b7d/1

== system case5/AC_1/d_iq_load_9_block ==
  note: d_iq_load_9 in case5
      | $1422.06408334706\,\mathrm{vq}_{\mathrm{bus},9}-902.564002881027\,\mathrm{iq}_{\mathrm{load},9}-376.991118430775\,\mathrm{id}_{\mathrm{load},9}$
      | Automatically generated on 2025-10-31 19:14:11 .
  State_id_load_9_b9788 : Inport
  State_iq_load_9_0cd3a : Inport  Port=2
  State_vq_bus_9_617f4 : Inport  Port=3
  Add_1dcdb : Sum
  Constant_-376.991118430775_61b84 : Constant  Value=-376.991118430775
  Constant_1422.06408334706_05b74 : Constant  Value=1422.06408334706
  Constant_902.564002881027_df512 : Constant  Value=902.564002881027
  Product_50b9d : Product
  Product_7109a : Product
  Product_b06d2 : Product
  Subtract_58088 : Sum  Inputs=+-
  Blockout_d_iq_load_9_aa725 : Outport
  wires:
  Constant_-376.991118430775_61b84/1 -> Product_b06d2/1
  Product_7109a/1 -> Subtract_58088/2
  State_id_load_9_b9788/1 -> Product_b06d2/2
  Add_1dcdb/1 -> Blockout_d_iq_load_9_aa725/1
  Constant_902.564002881027_df512/1 -> Product_7109a/1
  Product_50b9d/1 -> Add_1dcdb/2
  Product_b06d2/1 -> Subtract_58088/1
  State_iq_load_9_0cd3a/1 -> Product_7109a/2
  Constant_1422.06408334706_05b74/1 -> Product_50b9d/1
  State_vq_bus_9_617f4/1 -> Product_50b9d/2
  Subtract_58088/1 -> Add_1dcdb/1

== system case5/AC_1/d_vd_bus_1_block ==
  note: d_vd_bus_1 in case5
      | $37699111.8430775\,\mathrm{id}_{\mathrm{bus},1}+376.991118430775\,\mathrm{vq}_{\mathrm{bus},1}$
      | Automatically generated on 2025-10-31 19:13:44 .
  Alge_id_bus_1_8840e : Inport
  State_vq_bus_1_c0d62 : Inport  Port=2
  Add_cc81f : Sum
  Constant_376.991118430775_b99e0 : Constant  Value=376.991118430775
  Constant_37699111.8430775_ae00b : Constant  Value=37699111.8430775
  Product_b22d9 : Product
  Product_c7319 : Product
  Blockout_d_vd_bus_1_cb049 : Outport
  wires:
  Constant_37699111.8430775_ae00b/1 -> Product_b22d9/1
  Product_c7319/1 -> Add_cc81f/2
  Alge_id_bus_1_8840e/1 -> Product_b22d9/2
  Constant_376.991118430775_b99e0/1 -> Product_c7319/1
  State_vq_bus_1_c0d62/1 -> Product_c7319/2
  Add_cc81f/1 -> Blockout_d_vd_bus_1_cb049/1
  Product_b22d9/1 -> Add_cc81f/1

== system case5/AC_1/d_vd_bus_2_block ==
  note: d_vd_bus_2 in case5
      | $37699111.8430775\,\mathrm{id}_{\mathrm{bus},2}+376.991118430775\,\mathrm{vq}_{\mathrm{bus},2}$
      | Automatically generated on 2025-10-31 19:13:46 .
  Alge_id_bus_2_9f42b : Inport
  State_vq_bus_2_626a1 : Inport  Port=2
  Add_4db2f : Sum
  Constant_376.991118430775_f8b9e : Constant  Value=376.991118430775
  Constant_37699111.8430775_59018 : Constant  Value=37699111.8430775
  Product_0720a : Product
  Product_2f2a2 : Product
  Blockout_d_vd_bus_2_1e6bd : Outport
  wires:
  Constant_37699111.8430775_59018/1 -> Product_2f2a2/1
  Product_0720a/1 -> Add_4db2f/2
  Alge_id_bus_2_9f42b/1 -> Product_2f2a2/2
  Constant_376.991118430775_f8b9e/1 -> Product_0720a/1
  Product_2f2a2/1 -> Add_4db2f/1
  State_vq_bus_2_626a1/1 -> Product_0720a/2
  Add_4db2f/1 -> Blockout_d_vd_bus_2_1e6bd/1

== system case5/AC_1/d_vd_bus_3_block ==
  note: d_vd_bus_3 in case5
      | $37699111.8430775\,\mathrm{id}_{\mathrm{bus},3}+376.991118430775\,\mathrm{vq}_{\mathrm{bus},3}$
      | Automatically generated on 2025-10-31 19:13:48 .
  Alge_id_bus_3_04cef : Inport
  State_vq_bus_3_406ee : Inport  Port=2
  Add_c773f : Sum
  Constant_376.991118430775_da394 : Constant  Value=376.991118430775
  Constant_37699111.8430775_44b53 : Constant  Value=37699111.8430775
  Product_b3372 : Product
  Product_fc82d : Product
  Blockout_d_vd_bus_3_3d9b3 : Outport
  wires:
  Constant_37699111.8430775_44b53/1 -> Product_fc82d/1
  Product_b3372/1 -> Add_c773f/2
  Alge_id_bus_3_04cef/1 -> Product_fc82d/2
  Constant_376.991118430775_da394/1 -> Product_b3372/1
  Product_fc82d/1 -> Add_c773f/1
  State_vq_bus_3_406ee/1 -> Product_b3372/2
  Add_c773f/1 -> Blockout_d_vd_bus_3_3d9b3/1

== system case5/AC_1/d_vd_bus_4_block ==
  note: d_vd_bus_4 in case5
      | $2257.43184689087\,\mathrm{id}_{\mathrm{bus},4}+376.991118430775\,\mathrm{vq}_{\mathrm{bus},4}$
      | Automatically generated on 2025-10-31 19:13:50 .
  Alge_id_bus_4_3c99c : Inport
  State_vq_bus_4_56f16 : Inport  Port=2
  Add_19c35 : Sum
  Constant_2257.43184689087_cfe50 : Constant  Value=2257.43184689087
  Constant_376.991118430775_9d841 : Constant  Value=376.991118430775
  Product_222b3 : Product
  Product_3c6f5 : Product
  Blockout_d_vd_bus_4_f5d06 : Outport
  wires:
  Constant_2257.43184689087_cfe50/1 -> Product_222b3/1
  Product_3c6f5/1 -> Add_19c35/2
  Alge_id_bus_4_3c99c/1 -> Product_222b3/2
  Constant_376.991118430775_9d841/1 -> Product_3c6f5/1
  Product_222b3/1 -> Add_19c35/1
  State_vq_bus_4_56f16/1 -> Product_3c6f5/2
  Add_19c35/1 -> Blockout_d_vd_bus_4_f5d06/1

== system case5/AC_1/d_vd_bus_5_block ==
  note: d_vd_bus_5 in case5
      | $1461.2058853906\,\mathrm{id}_{\mathrm{bus},5}+376.991118430775\,\mathrm{vq}_{\mathrm{bus},5}$
      | Automatically generated on 2025-10-31 19:13:53 .
  Alge_id_bus_5_8ca73 : Inport
  State_vq_bus_5_14cdd : Inport  Port=2
  Add_b659c : Sum
  Constant_1461.2058853906_6856c : Constant  Value=1461.2058853906
  Constant_376.991118430775_d4960 : Constant  Value=376.991118430775
  Product_05bb8 : Product
  Product_fa143 : Product
  Blockout_d_vd_bus_5_8454f : Outport
  wires:
  Constant_1461.2058853906_6856c/1 -> Product_fa143/1
  Product_05bb8/1 -> Add_b659c/2
  Alge_id_bus_5_8ca73/1 -> Product_fa143/2
  Constant_376.991118430775_d4960/1 -> Product_05bb8/1
  Product_fa143/1 -> Add_b659c/1
  State_vq_bus_5_14cdd/1 -> Product_05bb8/2
  Add_b659c/1 -> Blockout_d_vd_bus_5_8454f/1

== system case5/AC_1/d_vd_bus_6_block ==
  note: d_vd_bus_6 in case5
      | $1329.77466818616\,\mathrm{id}_{\mathrm{bus},6}+376.991118430775\,\mathrm{vq}_{\mathrm{bus},6}$
      | Automatically generated on 2025-10-31 19:13:55 .
  Alge_id_bus_6_4022d : Inport
  State_vq_bus_6_3b173 : Inport  Port=2
  Add_15f4e : Sum
  Constant_1329.77466818616_0bbaa : Constant  Value=1329.77466818616
  Constant_376.991118430775_82588 : Constant  Value=376.991118430775
  Product_4fc2a : Product
  Product_a4cce : Product
  Blockout_d_vd_bus_6_37b4b : Outport
  wires:
  Constant_1329.77466818616_0bbaa/1 -> Product_a4cce/1
  Product_4fc2a/1 -> Add_15f4e/2
  Alge_id_bus_6_4022d/1 -> Product_a4cce/2
  Constant_376.991118430775_82588/1 -> Product_4fc2a/1
  Product_a4cce/1 -> Add_15f4e/1
  State_vq_bus_6_3b173/1 -> Product_4fc2a/2
  Add_15f4e/1 -> Blockout_d_vd_bus_6_37b4b/1

== system case5/AC_1/d_vd_bus_7_block ==
  note: d_vd_bus_7 in case5
      | $2106.09563369148\,\mathrm{id}_{\mathrm{bus},7}+376.991118430775\,\mathrm{vq}_{\mathrm{bus},7}$
      | Automatically generated on 2025-10-31 19:13:57 .
  Alge_id_bus_7_c0ece : Inport
  State_vq_bus_7_b7f85 : Inport  Port=2
  Add_ed5d5 : Sum
  Constant_2106.09563369148_4c5f3 : Constant  Value=2106.09563369148
  Constant_376.991118430775_2fc84 : Constant  Value=376.991118430775
  Product_130a4 : Product
  Product_c13fd : Product
  Blockout_d_vd_bus_7_c07fa : Outport
  wires:
  Constant_2106.09563369148_4c5f3/1 -> Product_130a4/1
  Product_c13fd/1 -> Add_ed5d5/2
  Alge_id_bus_7_c0ece/1 -> Product_130a4/2
  Constant_376.991118430775_2fc84/1 -> Product_c13fd/1
  Product_130a4/1 -> Add_ed5d5/1
  State_vq_bus_7_b7f85/1 -> Product_c13fd/2
  Add_ed5d5/1 -> Blockout_d_vd_bus_7_c07fa/1

== system case5/AC_1/d_vd_bus_8_block ==
  note: d_vd_bus_8 in case5
      | $1657.10381727813\,\mathrm{id}_{\mathrm{bus},8}+376.991118430775\,\mathrm{vq}_{\mathrm{bus},8}$
      | Automatically generated on 2025-10-31 19:13:59 .
  Alge_id_bus_8_d2bcb : Inport
  State_vq_bus_8_c6552 : Inport  Port=2
  Add_1b218 : Sum
  Constant_1657.10381727813_dd472 : Constant  Value=1657.10381727813
  Constant_376.991118430775_b3a5e : Constant  Value=376.991118430775
  Product_5337a : Product
  Product_a5bb4 : Product
  Blockout_d_vd_bus_8_47c26 : Outport
  wires:
  Constant_1657.10381727813_dd472/1 -> Product_a5bb4/1
  Product_5337a/1 -> Add_1b218/2
  Alge_id_bus_8_d2bcb/1 -> Product_a5bb4/2
  Constant_376.991118430775_b3a5e/1 -> Product_5337a/1
  Product_a5bb4/1 -> Add_1b218/1
  State_vq_bus_8_c6552/1 -> Product_5337a/2
  Add_1b218/1 -> Blockout_d_vd_bus_8_47c26/1

== system case5/AC_1/d_vd_bus_9_block ==
  note: d_vd_bus_9 in case5
      | $1564.27849971276\,\mathrm{id}_{\mathrm{bus},9}+376.991118430775\,\mathrm{vq}_{\mathrm{bus},9}$
      | Automatically generated on 2025-10-31 19:14:01 .
  Alge_id_bus_9_7e67e : Inport
  State_vq_bus_9_1df90 : Inport  Port=2
  Add_b904a : Sum
  Constant_1564.27849971276_387c5 : Constant  Value=1564.27849971276
  Constant_376.991118430775_1de93 : Constant  Value=376.991118430775
  Product_46e19 : Product
  Product_de015 : Product
  Blockout_d_vd_bus_9_48b9f : Outport
  wires:
  Constant_1564.27849971276_387c5/1 -> Product_de015/1
  Product_46e19/1 -> Add_b904a/2
  Alge_id_bus_9_7e67e/1 -> Product_de015/2
  Constant_376.991118430775_1de93/1 -> Product_46e19/1
  Product_de015/1 -> Add_b904a/1
  State_vq_bus_9_1df90/1 -> Product_46e19/2
  Add_b904a/1 -> Blockout_d_vd_bus_9_48b9f/1

== system case5/AC_1/d_vq_bus_1_block ==
  note: d_vq_bus_1 in case5
      | $37699111.8430775\,\mathrm{iq}_{\mathrm{bus},1}-376.991118430775\,\mathrm{vd}_{\mathrm{bus},1}$
      | Automatically generated on 2025-10-31 19:13:45 .
  Alge_iq_bus_1_bc35c : Inport
  State_vd_bus_1_e6515 : Inport  Port=2
  Constant_376.991118430775_4aeed : Constant  Value=376.991118430775
  Constant_37699111.8430775_32bb2 : Constant  Value=37699111.8430775
  Product_62fde : Product
  Product_73fbf : Product
  Subtract_74c44 : Sum  Inputs=+-
  Blockout_d_vq_bus_1_c9ee7 : Outport
  wires:
  Constant_37699111.8430775_32bb2/1 -> Product_62fde/1
  Constant_376.991118430775_4aeed/1 -> Product_73fbf/1
  Alge_iq_bus_1_bc35c/1 -> Product_62fde/2
  State_vd_bus_1_e6515/1 -> Product_73fbf/2
  Product_62fde/1 -> Subtract_74c44/1
  Product_73fbf/1 -> Subtract_74c44/2
  Subtract_74c44/1 -> Blockout_d_vq_bus_1_c9ee7/1

== system case5/AC_1/d_vq_bus_2_block ==
  note: d_vq_bus_2 in case5
      | $37699111.8430775\,\mathrm{iq}_{\mathrm{bus},2}-376.991118430775\,\mathrm{vd}_{\mathrm{bus},2}$
      | Automatically generated on 2025-10-31 19:13:47 .
  Alge_iq_bus_2_b4b58 : Inport
  State_vd_bus_2_003ed : Inport  Port=2
  Constant_376.991118430775_0ef0c : Constant  Value=376.991118430775
  Constant_37699111.8430775_42b1e : Constant  Value=37699111.8430775
  Product_5e177 : Product
  Product_d5909 : Product
  Subtract_fa8fe : Sum  Inputs=+-
  Blockout_d_vq_bus_2_8d2c4 : Outport
  wires:
  Constant_37699111.8430775_42b1e/1 -> Product_d5909/1
  Constant_376.991118430775_0ef0c/1 -> Product_5e177/1
  Alge_iq_bus_2_b4b58/1 -> Product_d5909/2
  State_vd_bus_2_003ed/1 -> Product_5e177/2
  Product_d5909/1 -> Subtract_fa8fe/1
  Product_5e177/1 -> Subtract_fa8fe/2
  Subtract_fa8fe/1 -> Blockout_d_vq_bus_2_8d2c4/1

== system case5/AC_1/d_vq_bus_3_block ==
  note: d_vq_bus_3 in case5
      | $37699111.8430775\,\mathrm{iq}_{\mathrm{bus},3}-376.991118430775\,\mathrm{vd}_{\mathrm{bus},3}$
      | Automatically generated on 2025-10-31 19:13:49 .
  Alge_iq_bus_3_7b7af : Inport
  State_vd_bus_3_f2360 : Inport  Port=2
  Constant_376.991118430775_d51c7 : Constant  Value=376.991118430775
  Constant_37699111.8430775_96700 : Constant  Value=37699111.8430775
  Product_32e1d : Product
  Product_e8cca : Product
  Subtract_2f895 : Sum  Inputs=+-
  Blockout_d_vq_bus_3_ffd35 : Outport
  wires:
  Constant_37699111.8430775_96700/1 -> Product_e8cca/1
  Constant_376.991118430775_d51c7/1 -> Product_32e1d/1
  Alge_iq_bus_3_7b7af/1 -> Product_e8cca/2
  State_vd_bus_3_f2360/1 -> Product_32e1d/2
  Product_e8cca/1 -> Subtract_2f895/1
  Product_32e1d/1 -> Subtract_2f895/2
  Subtract_2f895/1 -> Blockout_d_vq_bus_3_ffd35/1

== system case5/AC_1/d_vq_bus_4_block ==
  note: d_vq_bus_4 in case5
      | $2257.43184689087\,\mathrm{iq}_{\mathrm{bus},4}-376.991118430775\,\mathrm{vd}_{\mathrm{bus},4}$
      | Automatically generated on 2025-10-31 19:13:52 .
  Alge_iq_bus_4_d306c : Inport
  State_vd_bus_4_b3884 : Inport  Port=2
  Constant_2257.43184689087_0a839 : Constant  Value=2257.43184689087
  Constant_376.991118430775_9c638 : Constant  Value=376.991118430775
  Product_3a6df : Product
  Product_ca748 : Product
  Subtract_999dd : Sum  Inputs=+-
  Blockout_d_vq_bus_4_4979a : Outport
  wires:
  Constant_2257.43184689087_0a839/1 -> Product_3a6df/1
  Constant_376.991118430775_9c638/1 -> Product_ca748/1
  Alge_iq_bus_4_d306c/1 -> Product_3a6df/2
  State_vd_bus_4_b3884/1 -> Product_ca748/2
  Product_3a6df/1 -> Subtract_999dd/1
  Product_ca748/1 -> Subtract_999dd/2
  Subtract_999dd/1 -> Blockout_d_vq_bus_4_4979a/1

== system case5/AC_1/d_vq_bus_5_block ==
  note: d_vq_bus_5 in case5
      | $1461.2058853906\,\mathrm{iq}_{\mathrm{bus},5}-376.991118430775\,\mathrm{vd}_{\mathrm{bus},5}$
      | Automatically generated on 2025-10-31 19:13:54 .
  Alge_iq_bus_5_3167d : Inport
  State_vd_bus_5_f0a26 : Inport  Port=2
  Constant_1461.2058853906_8dd54 : Constant  Value=1461.2058853906
  Constant_376.991118430775_2b223 : Constant  Value=376.991118430775
  Product_255de : Product
  Product_d7383 : Product
  Subtract_20138 : Sum  Inputs=+-
  Blockout_d_vq_bus_5_9d8bd : Outport
  wires:
  Constant_1461.2058853906_8dd54/1 -> Product_d7383/1
  Constant_376.991118430775_2b223/1 -> Product_255de/1
  Alge_iq_bus_5_3167d/1 -> Product_d7383/2
  State_vd_bus_5_f0a26/1 -> Product_255de/2
  Product_d7383/1 -> Subtract_20138/1
  Product_255de/1 -> Subtract_20138/2
  Subtract_20138/1 -> Blockout_d_vq_bus_5_9d8bd/1

== system case5/AC_1/d_vq_bus_6_block ==
  note: d_vq_bus_6 in case5
      | $1329.77466818616\,\mathrm{iq}_{\mathrm{bus},6}-376.991118430775\,\mathrm{vd}_{\mathrm{bus},6}$
      | Automatically generated on 2025-10-31 19:13:56 .
  Alge_iq_bus_6_9948a : Inport
  State_vd_bus_6_96a25 : Inport  Port=2
  Constant_1329.77466818616_bf661 : Constant  Value=1329.77466818616
  Constant_376.991118430775_c8d89 : Constant  Value=376.991118430775
  Product_38b9b : Product
  Product_b549d : Product
  Subtract_a5ed0 : Sum  Inputs=+-
  Blockout_d_vq_bus_6_aa0b1 : Outport
  wires:
  Constant_1329.77466818616_bf661/1 -> Product_38b9b/1
  Constant_376.991118430775_c8d89/1 -> Product_b549d/1
  Alge_iq_bus_6_9948a/1 -> Product_38b9b/2
  State_vd_bus_6_96a25/1 -> Product_b549d/2
  Product_38b9b/1 -> Subtract_a5ed0/1
  Product_b549d/1 -> Subtract_a5ed0/2
  Subtract_a5ed0/1 -> Blockout_d_vq_bus_6_aa0b1/1
